simulink model "SMCC_Example_Controller"  (R2019a)
settings: Solver=FixedStepDiscrete  StartTime=0.0  StopTime=inf  FixedStep=Ts  RelTol=1e-3
values from neighbouring files (symbols this model uses):
  directions = obj.DirectionsInternal    [HelperPathAnalyzer.m]
undefined symbols (not defined in the file or in its folder): curvatures, speedProfile, Ts, Waypoints
libraries: drivingvehiclecontroller x2, drivinglib x1
settings Model: Creator=The MathWorks, Inc.  LastModifiedBy=allenkim
settings DataIOCC: SaveOutput=off  SaveTime=off  ReturnWorkspaceOutputs=off
settings OptimizationCC: DefaultParameterBehavior=Inlined  DefaultUnderspecifiedDataType=single  EnhancedBackFolding=on  PassReuseOutputArgsAs=Individual arguments  OptimizeBlockOrder=speed  DifferentSizesBufferReuse=on  OptimizationCustomize=off
settings DebuggingCC: ParameterPrecisionLossMsg=none  ParameterTunabilityLossMsg=error  PregeneratedLibrarySubsystemCodeDiagnostic=none  ArithmeticOperatorsInVariantConditions=warning
settings HardwareCC: ProdLongLongMode=on
settings SFSimCC: SimUseLocalCustomCode=off  MATLABDynamicMemAlloc=off
settings RTWCC: SystemTargetFile=ert.tlc  TemplateMakefile=ert_default_tmf  GenerateReport=on  RTWUseLocalCustomCode=off  BuildConfiguration=Faster Runs  IncludeHyperlinkInReport=on  LaunchReport=on  TargetLang=C++  GenerateTraceInfo=on  GenerateTraceReport=on  GenerateTraceReportSl=on  GenerateTraceReportSf=on  GenerateTraceReportEml=on
settings CodeAppCC: ForceParamTrailComments=on  IgnoreCustomStorageClasses=off  MaxIdLength=63  OperatorAnnotations=on  SimulinkDataObjDesc=on  SFDataObjDesc=on  CustomSymbolStrFcn=$N$M$F  InsertBlockDesc=on
settings ERTTargetCC: TargetLangStandard=C++03 (ISO)  GenerateSampleERTMain=on  MultiInstanceERTCode=on  CodeInterfacePackaging=C++ class  InlinedParameterPlacement=NonHierarchical  RootIOFormat=Structure reference  ERTCustomFileTemplate=example_file_process.tlc

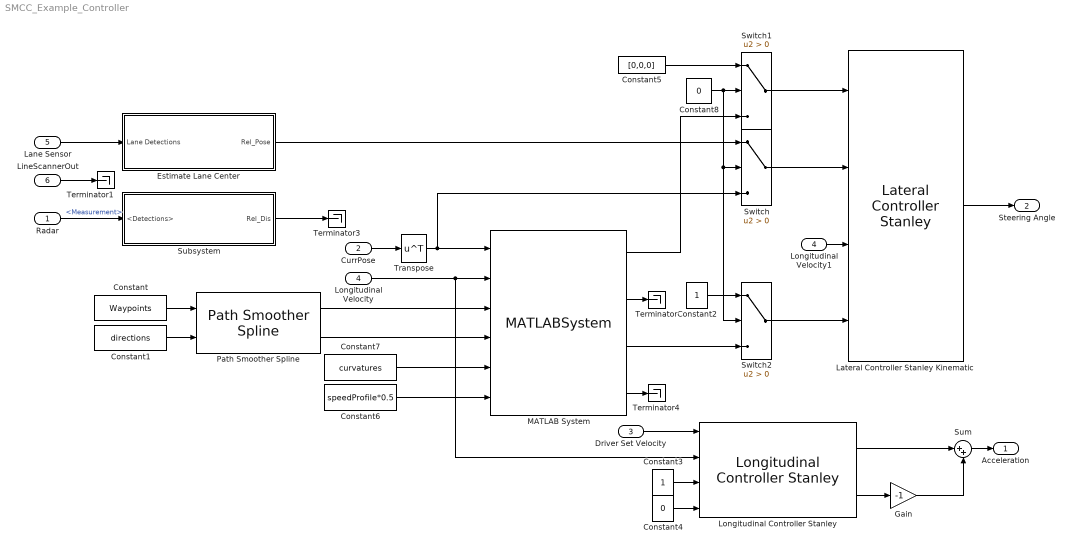
== system SMCC_Example_Controller ==
  Radar : Inport  OutDataTypeStr=Bus: BusRadar  PortDimensions=[1 1]  Interpolate=off  BusOutputAsStruct=on
  CurrPose : Inport  Port=2  OutDataTypeStr=double  Unit=m/s  PortDimensions=3  Interpolate=off
  Driver Set Velocity : Inport  Port=3  Interpolate=off
  Longitudinal Velocity : Inport  Port=4  OutDataTypeStr=double  Unit=m/s  Interpolate=off
  Lane Sensor : Inport  Port=5  OutDataTypeStr=Bus: LaneSensor  PortDimensions=[1 1]  Interpolate=off
  LineScannerOut : Inport  Port=6  OutDataTypeStr=double  PortDimensions=[5,2]  Interpolate=off
  Constant : Constant  Value=Waypoints  SampleTime=Ts
  Constant1 : Constant  Value=directions  SampleTime=Ts
  Constant2 : Constant
  Constant3 : Constant
  Constant4 : Constant  Value=0
  Constant5 : Constant  Value=[0,0,0]  SampleTime=Ts
  Constant6 : Constant  Value=speedProfile*0.5
  Constant7 : Constant  Value=curvatures
  Constant8 : Constant  Value=0
  Estimate Lane Center : Subsystem  TreatAsAtomicUnit=on  VariantControl=v2
      settings: RTWFileNameOpts=Use function name
  Gain : Gain  Gain=-1
  Lateral Controller Stanley Kinematic : drivingvehiclecontroller/Lateral Controller Stanley  VariantControl=Kinematic  ModelType=Kinematic bicycle model  PositionGainF=70  PositionGainR=0.01  YawRateGain=0.2  DelayGain=0.2  VehicleMass=1575  Lf=1.2  Lr=1.6  TireStiffness=19000  Wheelbase=wheelbase  MaxSteeringAngle=50
      settings: SourceProductName=Automated Driving Toolbox  SourceProductBaseCode=DR
  Longitudinal Controller Stanley : drivingvehiclecontroller/Longitudinal Controller Stanley  Kp=1  Ki=1  SampleTime=Ts  MaxAcceleration=0.5  MaxDeceleration=1
      settings: SourceProductName=Automated Driving Toolbox  SourceProductBaseCode=DR
  Longitudinal Velocity1 : InportShadow  Port=4  OutDataTypeStr=double  Unit=m/s  Interpolate=off
  MATLAB System : MATLABSystem  System=HelperPathAnalyzer  Wheelbase=wheelbase  HasResetOutput=off  SimulateUsing=Interpreted execution
      mask Type: HelperPathAnalyzer
      mask Display:
      | disp(['Helper' char(10) 'Path' char(10) 'Analyzer']);
      | port_label('input',1,'CurrPose');
      | port_label('input',2,'CurrVelocity');
      | port_label('input',3,'RefPoses');
      | port_label('input',4,'Directions');
      | port_label('input',5,'Curvatures');
      | port_label('input',6,'SpeedProfile');
      | port_label('output',1,'RefPose');
      | port_label('output',2,'RefVelocity');
      | port_label('output',3,'Direction');
      | port_label('output',4,'Curvature');
  Path Smoother Spline : drivinglib/Path Smoother Spline  NumSmoothPoses=500  MinSeparation=1e-3  SampleTime=-1  ShowOptionalOutports=off  SimulateUsing=Interpreted execution
      settings: SourceProductName=Automated Driving Toolbox  SourceProductBaseCode=DR
  Subsystem : Subsystem
  Sum : Sum  Inputs=|++
  Switch : Switch  Criteria=u2 > Threshold
  Switch1 : Switch  Criteria=u2 > Threshold
  Switch2 : Switch  Criteria=u2 > Threshold
  Terminator{,1,3..4} (4 alike) : Terminator
  Transpose : Math  Operator=transpose  SaturateOnIntegerOverflow=on
  Acceleration : Outport  PortDimensions=1
  Steering Angle : Outport  Port=2  PortDimensions=1
  wires:
  Lane Sensor/1 -> Estimate Lane Center/1(Lane Detections)
  Driver Set Velocity/1 -> Longitudinal Controller Stanley/1
  Sum/1 -> Acceleration/1
  CurrPose/1 -> Transpose/1
  Gain/1 -> Sum/2
  Longitudinal Controller Stanley/1 -> Sum/1
  Longitudinal Controller Stanley/2 -> Gain/1
  Subsystem/1(Rel_Dis) -> Terminator3/1
  Radar/1 -> Subsystem/1(<Detections>)  "<Measurement>"
  Longitudinal Velocity/1 -> Longitudinal Controller Stanley/2, MATLAB System/2
  Constant4/1 -> Longitudinal Controller Stanley/4
  Constant7/1 -> MATLAB System/5
  Path Smoother Spline/2 -> MATLAB System/4
  Constant6/1 -> MATLAB System/6
  Path Smoother Spline/1 -> MATLAB System/3
  MATLAB System/2 -> Terminator/1
  Estimate Lane Center/1(Rel_Pose) -> Switch/1
  Transpose/1 -> Switch/3, MATLAB System/1
  MATLAB System/4 -> Terminator4/1
  Lateral Controller Stanley Kinematic/1 -> Steering Angle/1
  Switch2/1 -> Lateral Controller Stanley Kinematic/4
  Constant3/1 -> Longitudinal Controller Stanley/3
  MATLAB System/3 -> Switch2/3
  Constant1/1 -> Path Smoother Spline/2
  Constant/1 -> Path Smoother Spline/1
  Constant8/1 -> Switch/2, Switch2/2, Switch1/2
  Switch/1 -> Lateral Controller Stanley Kinematic/2
  Switch1/1 -> Lateral Controller Stanley Kinematic/1
  MATLAB System/1 -> Switch1/3
  Constant5/1 -> Switch1/1
  Constant2/1 -> Switch2/1
  Longitudinal Velocity1/1 -> Lateral Controller Stanley Kinematic/3
  LineScannerOut/1 -> Terminator1/1

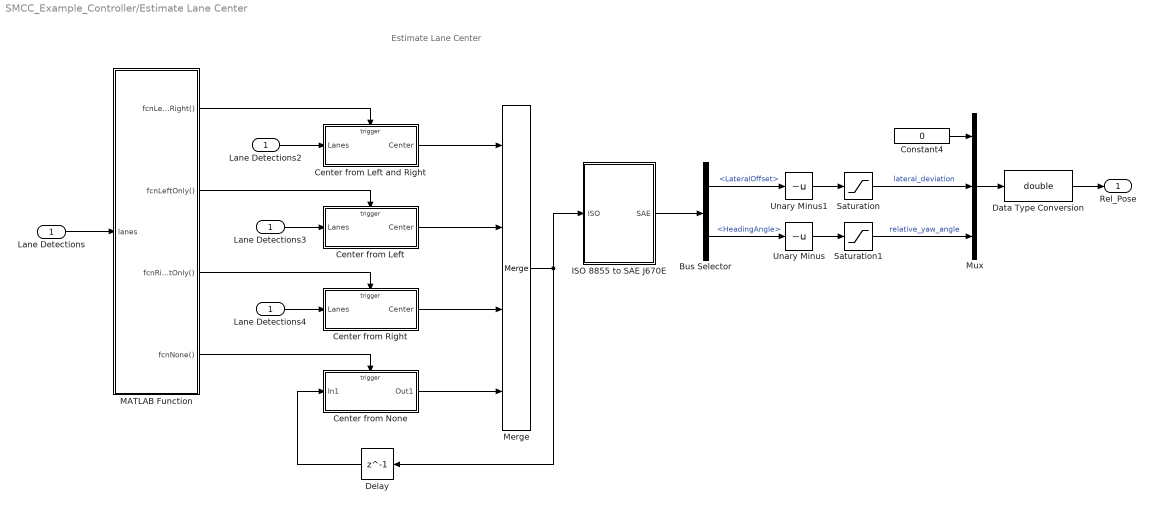
== system SMCC_Example_Controller/Estimate Lane Center ==
  note: Estimate Lane Center
  Lane Detections : Inport
  Bus Selector : BusSelector  OutputSignals=LateralOffset,HeadingAngle
  Center from Left : Subsystem  TreatAsAtomicUnit=on
  Center from Left and Right : Subsystem  TreatAsAtomicUnit=on
  Center from None : Subsystem  TreatAsAtomicUnit=on
  Center from Right : Subsystem  TreatAsAtomicUnit=on
  Constant4 : Constant  Value=0  OutDataTypeStr=single
  Data Type Conversion : DataTypeConversion  OutDataTypeStr=double
  Delay : Delay  DelayLength=1
  ISO 8855 to SAE J670E : Subsystem
  Lane Detections2 : InportShadow
  Lane Detections3 : InportShadow
  Lane Detections4 : InportShadow
  MATLAB Function : MATLAB Function  TreatAsAtomicUnit=on
  Merge : Merge  Inputs=4
  Mux : Mux  Inputs=3
  Saturation : Saturate
  Saturation1 : Saturate  UpperLimit=0.6  LowerLimit=-0.6
  Unary Minus : UnaryMinus
  Unary Minus1 : UnaryMinus
  Rel_Pose : Outport
  wires:
  Center from Right/1(Center) -> Merge/3
  Lane Detections3/1 -> Center from Left/1(Lanes)
  Lane Detections4/1 -> Center from Right/1(Lanes)
  MATLAB Function/2(fcnLeftOnly()) -> Center from Left/Trigger
  Center from None/1(Out1) -> Merge/4
  MATLAB Function/1(fcnLeftAndRight()) -> Center from Left and Right/Trigger
  Delay/1 -> Center from None/1(In1)
  Center from Left and Right/1(Center) -> Merge/1
  Lane Detections/1 -> MATLAB Function/1(lanes)
  Lane Detections2/1 -> Center from Left and Right/1(Lanes)
  MATLAB Function/3(fcnRightOnly()) -> Center from Right/Trigger
  MATLAB Function/4(fcnNone()) -> Center from None/Trigger
  Center from Left/1(Center) -> Merge/2
  Merge/1 -> ISO 8855 to SAE J670E/1(ISO), Delay/1
  Unary Minus/1 -> Saturation1/1
  Unary Minus1/1 -> Saturation/1
  Bus Selector/1 -> Unary Minus1/1  "<LateralOffset>"
  Bus Selector/2 -> Unary Minus/1  "<HeadingAngle>"
  ISO 8855 to SAE J670E/1(SAE) -> Bus Selector/1
  Constant4/1 -> Mux/1
  Saturation1/1 -> Mux/3  "relative_yaw_angle"
  Saturation/1 -> Mux/2  "lateral_deviation"
  Mux/1 -> Data Type Conversion/1
  Data Type Conversion/1 -> Rel_Pose/1

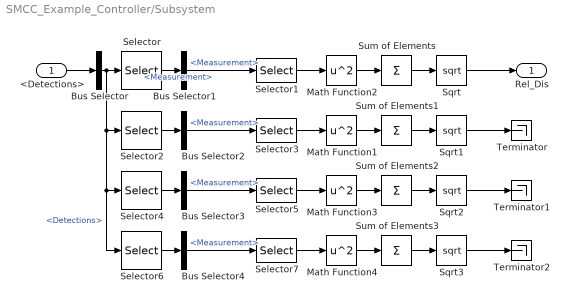
== system SMCC_Example_Controller/Subsystem ==
  <Detections> : Inport
  Bus Selector : BusSelector  OutputSignals=Detections
  Bus Selector{1..4} (4 alike) : BusSelector  OutputSignals=Measurement
  Math Function{1..4} (4 alike) : Math  Operator=square  SaturateOnIntegerOverflow=on
  Selector : Selector  InputPortWidth=10  IndexOptions=Index vector (dialog)  Indices=1  OutputSizes=1
  Selector{1,3,5,7} (4 alike) : Selector  InputPortWidth=6  IndexOptions=Index vector (dialog)  Indices=[1,2]  OutputSizes=1
  Selector2 : Selector  InputPortWidth=10  IndexOptions=Index vector (dialog)  Indices=2  OutputSizes=1
  Selector4 : Selector  InputPortWidth=10  IndexOptions=Index vector (dialog)  Indices=3  OutputSizes=1
  Selector6 : Selector  InputPortWidth=10  IndexOptions=Index vector (dialog)  Indices=4  OutputSizes=1
  Sqrt{,1..3} (4 alike) : Sqrt  SaturateOnIntegerOverflow=on
  Sum of Elements{,1..3} (4 alike) : Sum  Inputs=+
  Terminator : Terminator
  Terminator1 : Terminator
  Terminator2 : Terminator
  Rel_Dis : Outport
  wires:
  Selector1/1 -> Math Function2/1
  Bus Selector1/1 -> Selector1/1  "<Measurement>"
  Math Function2/1 -> Sum of Elements/1
  Sqrt/1 -> Rel_Dis/1
  <Detections>/1 -> Bus Selector/1
  Sum of Elements/1 -> Sqrt/1
  Selector/1 -> Bus Selector1/1  "<Measurement>"
  Bus Selector/1 -> Selector2/1, Selector6/1, Selector4/1, Selector/1  "<Detections>"
  Selector2/1 -> Bus Selector2/1
  Sum of Elements1/1 -> Sqrt1/1
  Sqrt1/1 -> Terminator/1
  Math Function1/1 -> Sum of Elements1/1
  Bus Selector2/1 -> Selector3/1  "<Measurement>"
  Selector3/1 -> Math Function1/1
  Selector5/1 -> Math Function3/1
  Bus Selector3/1 -> Selector5/1  "<Measurement>"
  Math Function3/1 -> Sum of Elements2/1
  Sqrt2/1 -> Terminator1/1
  Sum of Elements2/1 -> Sqrt2/1
  Selector4/1 -> Bus Selector3/1
  Selector6/1 -> Bus Selector4/1
  Sum of Elements3/1 -> Sqrt3/1
  Sqrt3/1 -> Terminator2/1
  Math Function4/1 -> Sum of Elements3/1
  Bus Selector4/1 -> Selector7/1  "<Measurement>"
  Selector7/1 -> Math Function4/1

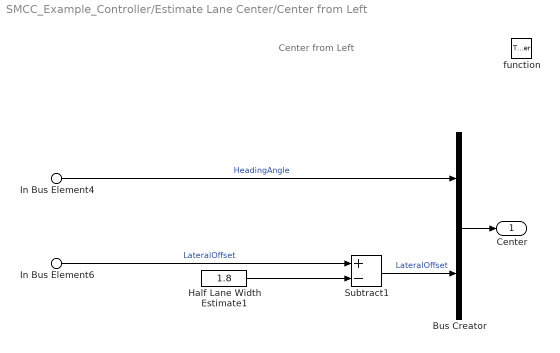
== system SMCC_Example_Controller/Estimate Lane Center/Center from Left ==
  note: Center from Left
  In Bus Element4 : Inport  PortName=Lanes  Element=Left.HeadingAngle
  In Bus Element6 : Inport  PortName=Lanes  Element=Left.LateralOffset
  function : TriggerPort  TriggerType=function-call  VariantControl=Variant
  Bus Creator : BusCreator  Inputs=2
  Half Lane Width Estimate1 : Constant  Value=1.8  OutDataTypeStr=Inherit: Inherit via back propagation
  Subtract1 : Sum  Inputs=+-
  Center : Outport
  wires:
  Half Lane Width Estimate1/1 -> Subtract1/2
  In Bus Element6/1 -> Subtract1/1  "LateralOffset"
  Subtract1/1 -> Bus Creator/2  "LateralOffset"
  In Bus Element4/1 -> Bus Creator/1  "HeadingAngle"
  Bus Creator/1 -> Center/1

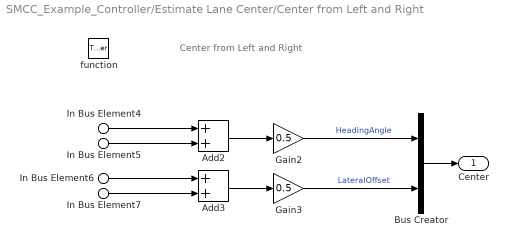
== system SMCC_Example_Controller/Estimate Lane Center/Center from Left and Right ==
  note: Center from Left and Right
  In Bus Element4 : Inport  PortName=Lanes  Element=Left.HeadingAngle
  In Bus Element6 : Inport  PortName=Lanes  Element=Left.LateralOffset
  In Bus Element5 : Inport  PortName=Lanes  Element=Right.HeadingAngle
  In Bus Element7 : Inport  PortName=Lanes  Element=Right.LateralOffset
  function : TriggerPort  TriggerType=function-call  VariantControl=Variant
  Add2 : Sum
  Add3 : Sum
  Bus Creator : BusCreator  Inputs=2
  Gain2 : Gain  Gain=0.5
  Gain3 : Gain  Gain=0.5
  Center : Outport
  wires:
  In Bus Element6/1 -> Add3/1
  In Bus Element7/1 -> Add3/2
  In Bus Element5/1 -> Add2/2
  In Bus Element4/1 -> Add2/1
  Bus Creator/1 -> Center/1
  Gain3/1 -> Bus Creator/2  "LateralOffset"
  Add3/1 -> Gain3/1
  Gain2/1 -> Bus Creator/1  "HeadingAngle"
  Add2/1 -> Gain2/1

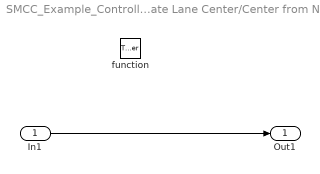
== system SMCC_Example_Controller/Estimate Lane Center/Center from None ==
  In1 : Inport
  function : TriggerPort  TriggerType=function-call  VariantControl=Variant
  Out1 : Outport
  wires:
  In1/1 -> Out1/1

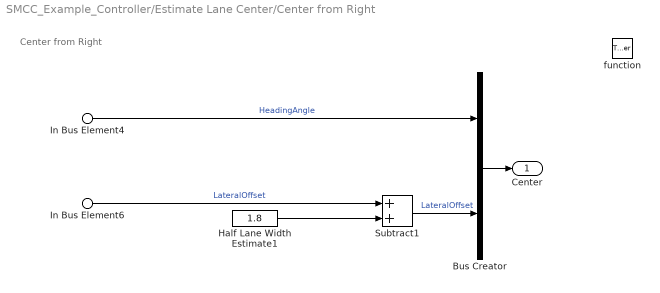
== system SMCC_Example_Controller/Estimate Lane Center/Center from Right ==
  note: Center from Right
  In Bus Element4 : Inport  PortName=Lanes  Element=Right.HeadingAngle
  In Bus Element6 : Inport  PortName=Lanes  Element=Right.LateralOffset
  function : TriggerPort  TriggerType=function-call  VariantControl=Variant
  Bus Creator : BusCreator  Inputs=2
  Half Lane Width Estimate1 : Constant  Value=1.8  OutDataTypeStr=Inherit: Inherit via back propagation
  Subtract1 : Sum
  Center : Outport
  wires:
  Bus Creator/1 -> Center/1
  Subtract1/1 -> Bus Creator/2  "LateralOffset"
  In Bus Element6/1 -> Subtract1/1  "LateralOffset"
  Half Lane Width Estimate1/1 -> Subtract1/2
  In Bus Element4/1 -> Bus Creator/1  "HeadingAngle"

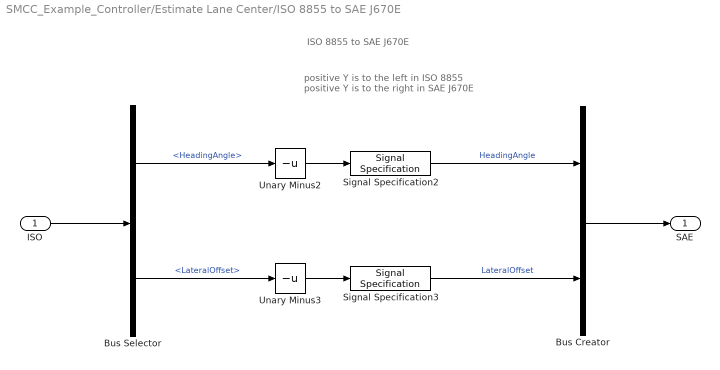
== system SMCC_Example_Controller/Estimate Lane Center/ISO 8855 to SAE J670E ==
  note: positive Y is to the left in ISO 8855
      | positive Y is to the right in SAE J670E
  note: ISO 8855 to SAE J670E
  ISO : Inport
  Bus Creator : BusCreator  Inputs=2
  Bus Selector : BusSelector  OutputSignals=HeadingAngle,LateralOffset
  Signal Specification2 : SignalSpecification  Unit=rad
  Signal Specification3 : SignalSpecification  Unit=m
  Unary Minus2 : UnaryMinus
  Unary Minus3 : UnaryMinus
  SAE : Outport
  wires:
  ISO/1 -> Bus Selector/1
  Bus Selector/1 -> Unary Minus2/1  "<HeadingAngle>"
  Bus Selector/2 -> Unary Minus3/1  "<LateralOffset>"
  Bus Creator/1 -> SAE/1
  Unary Minus2/1 -> Signal Specification2/1
  Unary Minus3/1 -> Signal Specification3/1
  Signal Specification2/1 -> Bus Creator/1  "HeadingAngle"
  Signal Specification3/1 -> Bus Creator/2  "LateralOffset"

== matlab function SMCC_Example_Controller/Estimate Lane Center/MATLAB Function ==
  data: lanes input
  events: fcnLeftAndRight output FUNCTION_CALL_EVENT; fcnLeftOnly output FUNCTION_CALL_EVENT; fcnRightOnly output FUNCTION_CALL_EVENT; fcnNone output FUNCTION_CALL_EVENT
function fcn(lanes)

leftStrength  = lanes.Left.Strength;
rightStrength = lanes.Right.Strength;

if (leftStrength > 0) && (rightStrength > 0)
   fcnLeftAndRight();
   
elseif leftStrength > 0
    fcnLeftOnly();
    
elseif rightStrength > 0
    fcnRightOnly();
    
else
    fcnNone();
end
